simulink model "L0508"  (Simulink 10.2)
settings: Solver=ode5  StartTime=0  StopTime=100  FixedStep=0.001  MaxStep=0.001  RelTol=1e-3
InitFcn:
  | LoadData
StopFcn:
  | PlotResult
values from neighbouring files (symbols this model uses):
  c = input('Damping parameter (10-1000 kg/s) c = ')    [LoadData.m]    (also in smdsys.m)
  hole_depth = 0.15    [LoadData.m]    (also in smdsys.m)
  k = input('Spring stiffness (50-5000 kg/s^2) k = ')    [LoadData.m]    (also in smdsys.m)
  m = 1000    [LoadData.m]    (also in smdsys.m)
  t1 = hole_start / v    (= 5)    [LoadData.m]    (also in smdsys.m)
  t2 = (hole_start + hole_length) / v    (= 5.05)    [LoadData.m]    (also in smdsys.m)
settings Model: Creator=Ranci  LastModifiedBy=Ranci
settings DataIOCC: SaveFormat=Dataset  SignalLoggingSaveFormat=Dataset  ReturnWorkspaceOutputs=on
settings OptimizationCC: LifeSpan=auto
settings DebuggingCC: UnderspecifiedInitializationDetection=Simplified  MergeDetectMultiDrivingBlocksExec=error  FcnCallInpInsideContextMsg=error  SFUnexpectedBacktrackingDiag=error  SFNoUnconditionalDefaultTransitionDiag=error  SFExecutionAtInitializationDiag=warning  ArithmeticOperatorsInVariantConditions=error
settings HardwareCC: ProdBitPerPointer=64  ProdBitPerSizeT=64  ProdBitPerPtrDiffT=64  ProdLargestAtomicFloat=Float  ProdIntDivRoundTo=Zero  ProdEndianess=LittleEndian  ProdWordSize=64  ProdHWDeviceType=Intel->x86-64 (Windows64)
settings ModelReferenceCC: PropagateSignalLabelsOutOfModel=on
settings SFSimCC: SimUseLocalCustomCode=on  CustomCodeUndefinedFunction=FilterOut
settings RTWCC: RTWUseLocalCustomCode=on
settings CodeAppCC: StateflowObjectComments=off
settings GRTTargetCC: TargetLangStandard=C99 (ISO)  CombineOutputUpdateFcns=on  GRTInterface=off
settings ConfigComp: CovMetricSettings=dwe  CovSaveCumulativeToWorkspaceVar=off  CovSaveSingleToWorkspaceVar=off  CovExternalEMLEnable=on

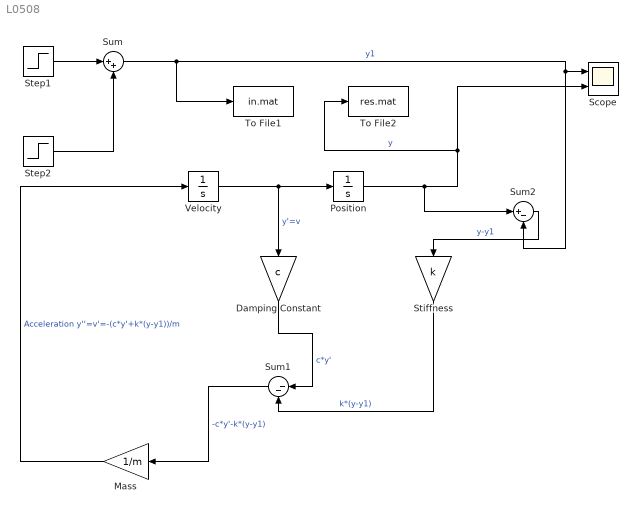
== system L0508 ==
  Damping Constant : Gain  Gain=c
  Mass : Gain  Gain=1/m
  Position : Integrator
  Scope : Scope  NumInputPorts=2
  Step1 : Step  Time=t1  After=-hole_depth  SampleTime=0.001
  Step2 : Step  Time=t2  After=hole_depth  SampleTime=0.001
  Stiffness : Gain  Gain=k
  Sum : Sum  Inputs=|++
  Sum1 : Sum  Inputs=|--
  Sum2 : Sum  Inputs=|+-
  To File1 : ToFile  Filename=in.mat  MatrixName=in  SaveFormat=Timeseries
  To File2 : ToFile  Filename=res.mat  MatrixName=res  SaveFormat=Timeseries
  Velocity : Integrator
  wires:
  Step1/1 -> Sum/1
  Step2/1 -> Sum/2
  Velocity/1 -> Damping Constant/1, Position/1  "y'=v"
  Damping Constant/1 -> Sum1/1  "c*y'"
  Sum1/1 -> Mass/1  "-c*y'-k*(y-y1)"
  Mass/1 -> Velocity/1  "Acceleration y''=v'=-(c*y'+k*(y-y1))/m"
  Position/1 -> To File2/1, Scope/2, Sum2/1  "y"
  Sum2/1 -> Stiffness/1  "y-y1"
  Stiffness/1 -> Sum1/2  "k*(y-y1)"
  Sum/1 -> To File1/1, Scope/1, Sum2/2  "y1"
